simulink library "INT_PhyMod_OpModeSelectNSync"  (R2016b)
settings: Solver=VariableStepAuto  StartTime=0.0  StopTime=10.0  RelTol=1e-3
settings Model: Creator=Administrator  LastModifiedBy=Administrator

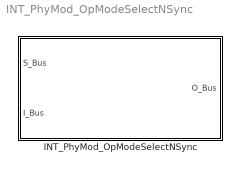
== system INT_PhyMod_OpModeSelectNSync ==
  INT_PhyMod_OpModeSelectNSync : Subsystem

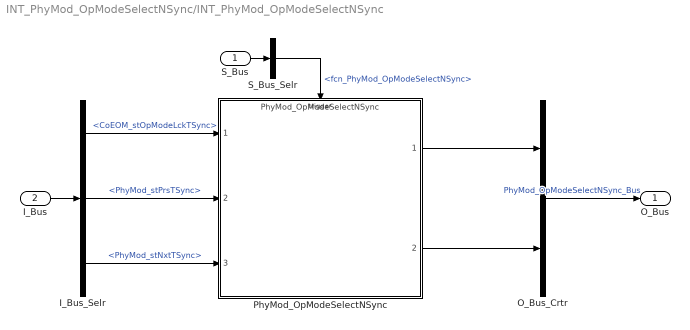
== system INT_PhyMod_OpModeSelectNSync/INT_PhyMod_OpModeSelectNSync ==
  S_Bus : Inport
  I_Bus : Inport  Port=2
  I_Bus_Selr : BusSelector  OutputSignals=CoEOM_stOpModeLckTSync,PhyMod_stPrsTSync,PhyMod_stNxtTSync
  O_Bus_Crtr : BusCreator  Inputs=2
  PhyMod_OpModeSelectNSync : ModelReference  ModelNameDialog=PhyMod_OpModeSelectNSync  ModelReferenceVersion=1.2  TriggerPortName=function  TriggerPortTriggerType=function-call  TriggerPortStatesWhenEnabling=held
  S_Bus_Selr : BusSelector  OutputSignals=fcn_PhyMod_OpModeSelectNSync
  O_Bus : Outport
  wires:
  S_Bus_Selr/1 -> PhyMod_OpModeSelectNSync/Trigger  "<fcn_PhyMod_OpModeSelectNSync>"
  S_Bus/1 -> S_Bus_Selr/1
  I_Bus/1 -> I_Bus_Selr/1
  I_Bus_Selr/1 -> PhyMod_OpModeSelectNSync/1  "<CoEOM_stOpModeLckTSync>"
  I_Bus_Selr/2 -> PhyMod_OpModeSelectNSync/2  "<PhyMod_stPrsTSync>"
  I_Bus_Selr/3 -> PhyMod_OpModeSelectNSync/3  "<PhyMod_stNxtTSync>"
  O_Bus_Crtr/1 -> O_Bus/1  "PhyMod_OpModeSelectNSync_Bus"
  PhyMod_OpModeSelectNSync/1 -> O_Bus_Crtr/1
  PhyMod_OpModeSelectNSync/2 -> O_Bus_Crtr/2
